simulink model "model_diag"  (R2024a)
settings: Solver=VariableStepAuto  StartTime=0.0  StopTime=10.0  RelTol=1e-3
settings Model: Creator=eva  LastModifiedBy=eva

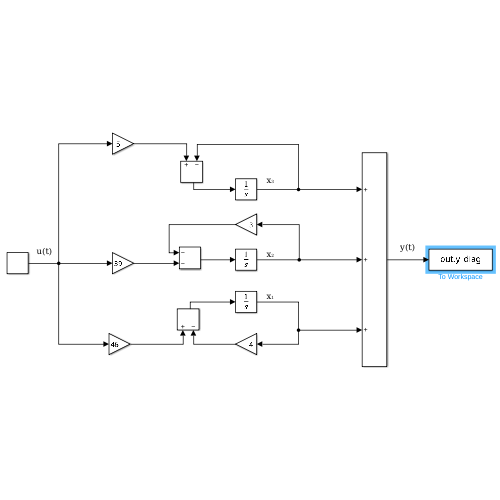
[thumbnail: Simulink's stored preview of the top-level diagram]
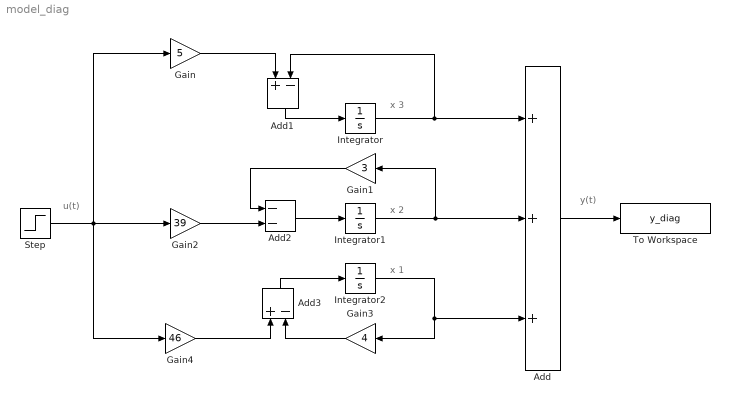
== system model_diag ==
  note: u(t)
  note: y(t)
  note: x 3
  note: x 2
  note: x 1
  Add : Sum  Inputs=+++
  Add1 : Sum  Inputs=+-
  Add2 : Sum  Inputs=--
  Add3 : Sum  Inputs=+-
  Gain : Gain  Gain=5
  Gain1 : Gain  Gain=3
  Gain2 : Gain  Gain=39
  Gain3 : Gain  Gain=4
  Gain4 : Gain  Gain=46
  Integrator : Integrator
  Integrator1 : Integrator
  Integrator2 : Integrator
  Step : Step  Time=0  SampleTime=0
  To Workspace : ToWorkspace  VariableName=y_diag  SaveFormat=Structure With Time  SampleTime=-1
  wires:
  Add/1 -> To Workspace/1
  Integrator/1 -> Add1/2, Add/1
  Integrator1/1 -> Gain1/1, Add/2
  Integrator2/1 -> Gain3/1, Add/3
  Add1/1 -> Integrator/1
  Step/1 -> Gain/1, Gain2/1, Gain4/1
  Gain/1 -> Add1/1
  Gain2/1 -> Add2/2
  Gain1/1 -> Add2/1
  Add2/1 -> Integrator1/1
  Add3/1 -> Integrator2/1
  Gain4/1 -> Add3/1
  Gain3/1 -> Add3/2
